simulink model "DR18E_Testpult"  (R2017a)
settings: Solver=ode1  StartTime=0.0  StopTime=Inf  FixedStep=0.001  RelTol=1e-3
PostLoadFcn:
  | , if any(exist('dsrtsu_mdlpostloadfcn', 'file') == [2, 3, 6]), try dsrtsu_mdlpostloadfcn('Execute', bdroot); catch fprintf('Error in PostLoadFcn (dsrtsu_mdlpostloadfcn) for model "%s":\n %s\n', bdroot, lasterr); end, end,
model workspace: external: MAT-File C:\Users\DeltaRacing\Documents\dSPACE\MABX_DR18E\Model\DR18E_MABX_Parameter.mat (data not in the file)
values from neighbouring files (symbols this model uses):
  am = 1/Ts    (= 1)    [DR18E_MABX_Parameter.m]
  bm = K/Ts    (= 0.05)    [DR18E_MABX_Parameter.m]
  cf = 41350    [DR18E_MABX_Parameter.m]
  cr = 41350    [DR18E_MABX_Parameter.m]
  Derating_HV_Battery_Kapa = 1    [DR18E_MABX_Parameter.m]
  Derating_Start_km = 16    [DR18E_MABX_Parameter.m]
  Drive_Mode = 0    [DR18E_MABX_Parameter.m]
  g = 1    [DR18E_MABX_Parameter.m]
  Gas_Modus = 2    [DR18E_MABX_Parameter.m]
  HV_Power_max = 80    [DR18E_MABX_Parameter.m]
  i_Getriebe = 3.3    [DR18E_MABX_Parameter.m]
  i_Lenkgetriebe = 4.32    [DR18E_MABX_Parameter.m]
  K_SET = 1    [DR18E_MABX_Parameter.m]
  Kapazitaet_HV_Battery_kWh = 6.6    [DR18E_MABX_Parameter.m]
  KW_T_Soll = 37    [DR18E_MABX_Parameter.m]
  lf = 1.2    [DR18E_MABX_Parameter.m]
  lr = 1.15    [DR18E_MABX_Parameter.m]
  m = mdriver + mvehicle    (= 310)    [DR18E_MABX_Parameter.m]
  M_max = 150    [DR18E_MABX_Parameter.m]
  Power_Limit_onoff = 0    [DR18E_MABX_Parameter.m]
  Reifenradius = 0.2351    [DR18E_MABX_Parameter.m]
  Strecke_Endu_km = 22    [DR18E_MABX_Parameter.m]
  TC_Decr_Gas = 0.00005    (= 5e-05)    [DR18E_MABX_Parameter.m]
  TC_Derivative = 0.4    [DR18E_MABX_Parameter.m]
  TC_Incr_Gas = 0.005    [DR18E_MABX_Parameter.m]
  TC_On = 0    [DR18E_MABX_Parameter.m]
  TC_Relay_Off = 0.065    [DR18E_MABX_Parameter.m]
  TC_Relay_On = 0.07    [DR18E_MABX_Parameter.m]
  TV_Mode = 2    [DR18E_MABX_Parameter.m]
  TV_On = 0    [DR18E_MABX_Parameter.m]
  TV_Override = 1    [DR18E_MABX_Parameter.m]
  y = 0.8    [DR18E_MABX_Parameter.m]
undefined symbols (not defined in the file or in its folder): D, DiscIntNeverNeededParam, I, K_OL, P
libraries: simulink x288, rtican x100, rtiusbflightreclib x40, rti1401lib_dio_type3 x10, simulink_extras x10, rti1401lib_adc_type4 x8, rti1401lib_II_base x7
(part 26 of 27)

== system DR18E_Testpult/Eingabe Fahrzeug/BMS/Voltage Stack 1-2/Voltage Stack 1/RX Timeout Detection2 ==
  RX status : Inport
  Timeout (n Samples) : Inport  Port=2
  Subsystem : Subsystem  TreatAsAtomicUnit=on
  Terminator_4 : Terminator
  RX Timeout Error : Outport
  wires:
  RX status/1 -> Subsystem/1(TXStatus)
  Subsystem/1(Rampe) -> Terminator_4/1
  Subsystem/2(RX Timeout Error) -> RX Timeout Error/1  "RX Timeout"
  Timeout (n Samples)/1 -> Subsystem/2(Timeout)

== system DR18E_Testpult/Eingabe Fahrzeug/BMS/Voltage Stack 1-2/Voltage Stack 2/RX Timeout Detection ==
  RX status : Inport
  Timeout (n Samples) : Inport  Port=2
  Subsystem : Subsystem  TreatAsAtomicUnit=on
  Terminator_4 : Terminator
  RX Timeout Error : Outport
  wires:
  RX status/1 -> Subsystem/1(TXStatus)
  Subsystem/1(Rampe) -> Terminator_4/1
  Subsystem/2(RX Timeout Error) -> RX Timeout Error/1  "RX Timeout"
  Timeout (n Samples)/1 -> Subsystem/2(Timeout)

== system DR18E_Testpult/Eingabe Fahrzeug/BMS/Voltage Stack 1-2/Voltage Stack 2/RX Timeout Detection1 ==
  RX status : Inport
  Timeout (n Samples) : Inport  Port=2
  Subsystem : Subsystem  TreatAsAtomicUnit=on
  Terminator_4 : Terminator
  RX Timeout Error : Outport
  wires:
  RX status/1 -> Subsystem/1(TXStatus)
  Subsystem/1(Rampe) -> Terminator_4/1
  Subsystem/2(RX Timeout Error) -> RX Timeout Error/1  "RX Timeout"
  Timeout (n Samples)/1 -> Subsystem/2(Timeout)

== system DR18E_Testpult/Eingabe Fahrzeug/BMS/Voltage Stack 1-2/Voltage Stack 2/RX Timeout Detection2 ==
  RX status : Inport
  Timeout (n Samples) : Inport  Port=2
  Subsystem : Subsystem  TreatAsAtomicUnit=on
  Terminator_4 : Terminator
  RX Timeout Error : Outport
  wires:
  RX status/1 -> Subsystem/1(TXStatus)
  Subsystem/1(Rampe) -> Terminator_4/1
  Subsystem/2(RX Timeout Error) -> RX Timeout Error/1  "RX Timeout"
  Timeout (n Samples)/1 -> Subsystem/2(Timeout)

== system DR18E_Testpult/Eingabe Fahrzeug/BMS/Voltage Stack 3-4/Voltage Stack 3/RX Timeout Detection ==
  RX status : Inport
  Timeout (n Samples) : Inport  Port=2
  Subsystem : Subsystem  TreatAsAtomicUnit=on
  Terminator_4 : Terminator
  RX Timeout Error : Outport
  wires:
  RX status/1 -> Subsystem/1(TXStatus)
  Subsystem/1(Rampe) -> Terminator_4/1
  Subsystem/2(RX Timeout Error) -> RX Timeout Error/1  "RX Timeout"
  Timeout (n Samples)/1 -> Subsystem/2(Timeout)

== system DR18E_Testpult/Eingabe Fahrzeug/BMS/Voltage Stack 3-4/Voltage Stack 3/RX Timeout Detection1 ==
  RX status : Inport
  Timeout (n Samples) : Inport  Port=2
  Subsystem : Subsystem  TreatAsAtomicUnit=on
  Terminator_4 : Terminator
  RX Timeout Error : Outport
  wires:
  RX status/1 -> Subsystem/1(TXStatus)
  Subsystem/1(Rampe) -> Terminator_4/1
  Subsystem/2(RX Timeout Error) -> RX Timeout Error/1  "RX Timeout"
  Timeout (n Samples)/1 -> Subsystem/2(Timeout)

== system DR18E_Testpult/Eingabe Fahrzeug/BMS/Voltage Stack 3-4/Voltage Stack 3/RX Timeout Detection2 ==
  RX status : Inport
  Timeout (n Samples) : Inport  Port=2
  Subsystem : Subsystem  TreatAsAtomicUnit=on
  Terminator_4 : Terminator
  RX Timeout Error : Outport
  wires:
  RX status/1 -> Subsystem/1(TXStatus)
  Subsystem/1(Rampe) -> Terminator_4/1
  Subsystem/2(RX Timeout Error) -> RX Timeout Error/1  "RX Timeout"
  Timeout (n Samples)/1 -> Subsystem/2(Timeout)

== system DR18E_Testpult/Eingabe Fahrzeug/BMS/Voltage Stack 3-4/Voltage Stack 4/RX Timeout Detection ==
  RX status : Inport
  Timeout (n Samples) : Inport  Port=2
  Subsystem : Subsystem  TreatAsAtomicUnit=on
  Terminator_4 : Terminator
  RX Timeout Error : Outport
  wires:
  RX status/1 -> Subsystem/1(TXStatus)
  Subsystem/1(Rampe) -> Terminator_4/1
  Subsystem/2(RX Timeout Error) -> RX Timeout Error/1  "RX Timeout"
  Timeout (n Samples)/1 -> Subsystem/2(Timeout)

== system DR18E_Testpult/Eingabe Fahrzeug/BMS/Voltage Stack 3-4/Voltage Stack 4/RX Timeout Detection1 ==
  RX status : Inport
  Timeout (n Samples) : Inport  Port=2
  Subsystem : Subsystem  TreatAsAtomicUnit=on
  Terminator_4 : Terminator
  RX Timeout Error : Outport
  wires:
  RX status/1 -> Subsystem/1(TXStatus)
  Subsystem/1(Rampe) -> Terminator_4/1
  Subsystem/2(RX Timeout Error) -> RX Timeout Error/1  "RX Timeout"
  Timeout (n Samples)/1 -> Subsystem/2(Timeout)

== system DR18E_Testpult/Eingabe Fahrzeug/BMS/Voltage Stack 3-4/Voltage Stack 4/RX Timeout Detection2 ==
  RX status : Inport
  Timeout (n Samples) : Inport  Port=2
  Subsystem : Subsystem  TreatAsAtomicUnit=on
  Terminator_4 : Terminator
  RX Timeout Error : Outport
  wires:
  RX status/1 -> Subsystem/1(TXStatus)
  Subsystem/1(Rampe) -> Terminator_4/1
  Subsystem/2(RX Timeout Error) -> RX Timeout Error/1  "RX Timeout"
  Timeout (n Samples)/1 -> Subsystem/2(Timeout)

== system DR18E_Testpult/Eingabe Fahrzeug/BMS/Voltage Stack 5-6/Voltage Stack 5/RX Timeout Detection ==
  RX status : Inport
  Timeout (n Samples) : Inport  Port=2
  Subsystem : Subsystem  TreatAsAtomicUnit=on
  Terminator_4 : Terminator
  RX Timeout Error : Outport
  wires:
  RX status/1 -> Subsystem/1(TXStatus)
  Subsystem/1(Rampe) -> Terminator_4/1
  Subsystem/2(RX Timeout Error) -> RX Timeout Error/1  "RX Timeout"
  Timeout (n Samples)/1 -> Subsystem/2(Timeout)

== system DR18E_Testpult/Eingabe Fahrzeug/BMS/Voltage Stack 5-6/Voltage Stack 5/RX Timeout Detection1 ==
  RX status : Inport
  Timeout (n Samples) : Inport  Port=2
  Subsystem : Subsystem  TreatAsAtomicUnit=on
  Terminator_4 : Terminator
  RX Timeout Error : Outport
  wires:
  RX status/1 -> Subsystem/1(TXStatus)
  Subsystem/1(Rampe) -> Terminator_4/1
  Subsystem/2(RX Timeout Error) -> RX Timeout Error/1  "RX Timeout"
  Timeout (n Samples)/1 -> Subsystem/2(Timeout)

== system DR18E_Testpult/Eingabe Fahrzeug/BMS/Voltage Stack 5-6/Voltage Stack 5/RX Timeout Detection2 ==
  RX status : Inport
  Timeout (n Samples) : Inport  Port=2
  Subsystem : Subsystem  TreatAsAtomicUnit=on
  Terminator_4 : Terminator
  RX Timeout Error : Outport
  wires:
  RX status/1 -> Subsystem/1(TXStatus)
  Subsystem/1(Rampe) -> Terminator_4/1
  Subsystem/2(RX Timeout Error) -> RX Timeout Error/1  "RX Timeout"
  Timeout (n Samples)/1 -> Subsystem/2(Timeout)

== system DR18E_Testpult/Eingabe Fahrzeug/BMS/Voltage Stack 5-6/Voltage Stack 6/RX Timeout Detection ==
  RX status : Inport
  Timeout (n Samples) : Inport  Port=2
  Subsystem : Subsystem  TreatAsAtomicUnit=on
  Terminator_4 : Terminator
  RX Timeout Error : Outport
  wires:
  RX status/1 -> Subsystem/1(TXStatus)
  Subsystem/1(Rampe) -> Terminator_4/1
  Subsystem/2(RX Timeout Error) -> RX Timeout Error/1  "RX Timeout"
  Timeout (n Samples)/1 -> Subsystem/2(Timeout)

== system DR18E_Testpult/Eingabe Fahrzeug/BMS/Voltage Stack 5-6/Voltage Stack 6/RX Timeout Detection1 ==
  RX status : Inport
  Timeout (n Samples) : Inport  Port=2
  Subsystem : Subsystem  TreatAsAtomicUnit=on
  Terminator_4 : Terminator
  RX Timeout Error : Outport
  wires:
  RX status/1 -> Subsystem/1(TXStatus)
  Subsystem/1(Rampe) -> Terminator_4/1
  Subsystem/2(RX Timeout Error) -> RX Timeout Error/1  "RX Timeout"
  Timeout (n Samples)/1 -> Subsystem/2(Timeout)

== system DR18E_Testpult/Eingabe Fahrzeug/BMS/Voltage Stack 5-6/Voltage Stack 6/RX Timeout Detection2 ==
  RX status : Inport
  Timeout (n Samples) : Inport  Port=2
  Subsystem : Subsystem  TreatAsAtomicUnit=on
  Terminator_4 : Terminator
  RX Timeout Error : Outport
  wires:
  RX status/1 -> Subsystem/1(TXStatus)
  Subsystem/1(Rampe) -> Terminator_4/1
  Subsystem/2(RX Timeout Error) -> RX Timeout Error/1  "RX Timeout"
  Timeout (n Samples)/1 -> Subsystem/2(Timeout)

== system DR18E_Testpult/Eingabe Fahrzeug/BMS/Voltage Stack 7-8/Voltage Stack 7/RX Timeout Detection ==
  RX status : Inport
  Timeout (n Samples) : Inport  Port=2
  Subsystem : Subsystem  TreatAsAtomicUnit=on
  Terminator_4 : Terminator
  RX Timeout Error : Outport
  wires:
  RX status/1 -> Subsystem/1(TXStatus)
  Subsystem/1(Rampe) -> Terminator_4/1
  Subsystem/2(RX Timeout Error) -> RX Timeout Error/1  "RX Timeout"
  Timeout (n Samples)/1 -> Subsystem/2(Timeout)

== system DR18E_Testpult/Eingabe Fahrzeug/BMS/Voltage Stack 7-8/Voltage Stack 7/RX Timeout Detection1 ==
  RX status : Inport
  Timeout (n Samples) : Inport  Port=2
  Subsystem : Subsystem  TreatAsAtomicUnit=on
  Terminator_4 : Terminator
  RX Timeout Error : Outport
  wires:
  RX status/1 -> Subsystem/1(TXStatus)
  Subsystem/1(Rampe) -> Terminator_4/1
  Subsystem/2(RX Timeout Error) -> RX Timeout Error/1  "RX Timeout"
  Timeout (n Samples)/1 -> Subsystem/2(Timeout)

== system DR18E_Testpult/Eingabe Fahrzeug/BMS/Voltage Stack 7-8/Voltage Stack 7/RX Timeout Detection2 ==
  RX status : Inport
  Timeout (n Samples) : Inport  Port=2
  Subsystem : Subsystem  TreatAsAtomicUnit=on
  Terminator_4 : Terminator
  RX Timeout Error : Outport
  wires:
  RX status/1 -> Subsystem/1(TXStatus)
  Subsystem/1(Rampe) -> Terminator_4/1
  Subsystem/2(RX Timeout Error) -> RX Timeout Error/1  "RX Timeout"
  Timeout (n Samples)/1 -> Subsystem/2(Timeout)

== system DR18E_Testpult/Eingabe Fahrzeug/BMS/Voltage Stack 7-8/Voltage Stack 8/RX Timeout Detection ==
  RX status : Inport
  Timeout (n Samples) : Inport  Port=2
  Subsystem : Subsystem  TreatAsAtomicUnit=on
  Terminator_4 : Terminator
  RX Timeout Error : Outport
  wires:
  RX status/1 -> Subsystem/1(TXStatus)
  Subsystem/1(Rampe) -> Terminator_4/1
  Subsystem/2(RX Timeout Error) -> RX Timeout Error/1  "RX Timeout"
  Timeout (n Samples)/1 -> Subsystem/2(Timeout)

== system DR18E_Testpult/Eingabe Fahrzeug/BMS/Voltage Stack 7-8/Voltage Stack 8/RX Timeout Detection1 ==
  RX status : Inport
  Timeout (n Samples) : Inport  Port=2
  Subsystem : Subsystem  TreatAsAtomicUnit=on
  Terminator_4 : Terminator
  RX Timeout Error : Outport
  wires:
  RX status/1 -> Subsystem/1(TXStatus)
  Subsystem/1(Rampe) -> Terminator_4/1
  Subsystem/2(RX Timeout Error) -> RX Timeout Error/1  "RX Timeout"
  Timeout (n Samples)/1 -> Subsystem/2(Timeout)

== system DR18E_Testpult/Eingabe Fahrzeug/BMS/Voltage Stack 7-8/Voltage Stack 8/RX Timeout Detection2 ==
  RX status : Inport
  Timeout (n Samples) : Inport  Port=2
  Subsystem : Subsystem  TreatAsAtomicUnit=on
  Terminator_4 : Terminator
  RX Timeout Error : Outport
  wires:
  RX status/1 -> Subsystem/1(TXStatus)
  Subsystem/1(Rampe) -> Terminator_4/1
  Subsystem/2(RX Timeout Error) -> RX Timeout Error/1  "RX Timeout"
  Timeout (n Samples)/1 -> Subsystem/2(Timeout)

== system DR18E_Testpult/Eingabe Fahrzeug/Inverter Feedback Messages/Istwerte Umrichter 1 empfangen /Drehzahl/PT1 Discrete2 ==
  u : Inport
  K : Inport  Port=2
  T : Inport  Port=3
  Memory : Memory
  Product : Product
  Product1 : Product
  Subsystem : Subsystem
  Sum : Sum  Inputs=|+-
  Sum1 : Sum  Inputs=|++
  y : Outport
  wires:
  K/1 -> Product/1
  Subsystem/1(T*) -> Product1/1
  u/1 -> Product/2
  Sum/1 -> Product1/2
  Product1/1 -> Sum1/1
  Memory/1 -> Sum1/2, Sum/2
  Sum1/1 -> y/1, Memory/1
  Product/1 -> Sum/1
  T/1 -> Subsystem/1(T)

== system DR18E_Testpult/Eingabe Fahrzeug/Inverter Feedback Messages/Istwerte Umrichter 1 empfangen /Drehzahl/Skalierung Drehzahl ==
  In1 : Inport
  Gain : Gain  Gain=4000/2^15
  Out1 : Outport
  wires:
  Gain/1 -> Out1/1
  In1/1 -> Gain/1

== system DR18E_Testpult/Eingabe Fahrzeug/Inverter Feedback Messages/Istwerte Umrichter 2 empfangen/Drehzahl/PT1 Discrete2 ==
  u : Inport
  K : Inport  Port=2
  T : Inport  Port=3
  Memory : Memory
  Product : Product
  Product1 : Product
  Subsystem : Subsystem
  Sum : Sum  Inputs=|+-
  Sum1 : Sum  Inputs=|++
  y : Outport
  wires:
  K/1 -> Product/1
  Subsystem/1(T*) -> Product1/1
  u/1 -> Product/2
  Sum/1 -> Product1/2
  Product1/1 -> Sum1/1
  Memory/1 -> Sum1/2, Sum/2
  Sum1/1 -> y/1, Memory/1
  Product/1 -> Sum/1
  T/1 -> Subsystem/1(T)

== system DR18E_Testpult/Eingabe Fahrzeug/Inverter Feedback Messages/Istwerte Umrichter 2 empfangen/Drehzahl/Skalierung Drehzahl ==
  In1 : Inport
  Gain : Gain  Gain=4000/(2^15)
  Out1 : Outport
  wires:
  In1/1 -> Gain/1
  Gain/1 -> Out1/1

== system DR18E_Testpult/Eingabe Fahrzeug/MicroAutoBox/AI/Umrechnung Widerstand - Temperatur NTC/PT1 Discrete1 ==
  u : Inport
  K : Inport  Port=2
  T : Inport  Port=3
  Memory : Memory
  Product : Product
  Product1 : Product
  Subsystem : Subsystem
  Sum : Sum  Inputs=|+-
  Sum1 : Sum  Inputs=|++
  y : Outport
  wires:
  K/1 -> Product/1
  Subsystem/1(T*) -> Product1/1
  u/1 -> Product/2
  Sum/1 -> Product1/2
  Product1/1 -> Sum1/1
  Memory/1 -> Sum1/2, Sum/2
  Sum1/1 -> y/1, Memory/1
  Product/1 -> Sum/1
  T/1 -> Subsystem/1(T)

== system DR18E_Testpult/Eingabe Fahrzeug/MicroAutoBox/AI/Umrechnung Widerstand - Temperatur NTC1/PT1 Discrete1 ==
  u : Inport
  K : Inport  Port=2
  T : Inport  Port=3
  Memory : Memory
  Product : Product
  Product1 : Product
  Subsystem : Subsystem
  Sum : Sum  Inputs=|+-
  Sum1 : Sum  Inputs=|++
  y : Outport
  wires:
  K/1 -> Product/1
  Subsystem/1(T*) -> Product1/1
  u/1 -> Product/2
  Sum/1 -> Product1/2
  Product1/1 -> Sum1/1
  Memory/1 -> Sum1/2, Sum/2
  Sum1/1 -> y/1, Memory/1
  Product/1 -> Sum/1
  T/1 -> Subsystem/1(T)

== system DR18E_Testpult/RTI Data/RTI Data Store/RTI Data Store/RTI Data Store/RTI Data Store ==

== system DR18E_Testpult/Verarbeitung/Bremse/PlausibilityCheck/PT1 Discrete1/Subsystem ==
  T : Inport
  Constant : Constant
  Constant2 : Constant
  Divide : Product  Inputs=*/
  Divide1 : Product  Inputs=*/
  Sum : Sum  Inputs=|++
  Weighted Sample Time : SampleTimeMath  TsampMathOp=Ts Only
  T* : Outport
  wires:
  Divide/1 -> T*/1
  Weighted Sample Time/1 -> Divide1/2
  Constant/1 -> Divide/1
  Sum/1 -> Divide/2
  T/1 -> Divide1/1
  Constant2/1 -> Sum/2
  Divide1/1 -> Sum/1

== system DR18E_Testpult/Verarbeitung/DR18E Torque Control/Derating/Derating_Strategie_Reichweite/Verbrauch_Wh//km ==
  In1 : Inport
  Data Type Conversion : DataTypeConversion
  Gain : Gain
  USB_FLIGHT_REC_BL1 : rtiusbflightreclib/USB_FLIGHT_REC_BL1  VarName=Verbrauch_Whprokm  DataType=Single  SampleTime=-1  TLCFileName=rtiusbflightrecwrite  Reserved1=[]  Reserved2=[]  Reserved3=[]  Reserved4=[]  DSProperties=struct('RTI',struct('Version',uint32(3),'BlockType',struct('isSLSource',uint8(0),'isSLSink',uint8(1),'isHWSource',uint8(0),'isHWSink',uint8(0),'isSetup',uint8(0),'isInline',uint8(1),'isNonInline',uint8(0),'isInterrupt',uint8(0),'isChannelwise',uint8(0)),'IOBoardType',{{'DSUSB','FLIGHTREC'}},'UnitType','FLIGHTREC','Identifier','WRITE','DialogType','SL','BlockSet','RTIUSBFLIGHTREC','SlaveProcessor','NONE'))  RTIBlockInterface=struct('InputPortsActive',1,'InputPortsWidth',int32(1),'InputPortsDataType',{{'SS_SINGLE'}},'BlockDisplay',{{['Write to\nUSB Flight Recorder'],'center'}},'IconTransparency','off','InitLevel',3,'BlockName',struct('Token',{{'USB_FLIGHT_REC_BL1'}}),'MaskDescription',['Write input to the Flight Recorder. Recorded data can be referenced by the specified variable.'],'SampleTime',{{-1}})  RTIBlockParameters=struct('VarName',{{'Verbrauch_Whprokm','OFF',[]}},'DataType',{{'Single','OFF',[]}},'SampleTime',{{-1,'OFF',[]}},'TLCFileName',{{'rtiusbflightrecwrite','OFF',[]}})  RTISFcnParameters=struct('VarName','char','DataType','char','SampleTime','double','TLCFileName','char')  RTIBlockParaDefault=struct('VarName','Var1','DataType','Single','SampleTime',-1,'TLCFileName','rtiusbflightrecwrite')
      settings: SourceProductName=dSPACE RTI USB Flight Rec Blockset
  wires:
  Data Type Conversion/1 -> USB_FLIGHT_REC_BL1/1
  In1/1 -> Gain/1
  Gain/1 -> Data Type Conversion/1

== system DR18E_Testpult/Verarbeitung/DR18E Torque Control/TV RL/TV DR17E/Drehmomentverteilung links//rechts ==
  DeltaM_in : Inport
  Gain links : Gain
  deltaM_Out : Outport
  wires:
  DeltaM_in/1 -> Gain links/1  "delta_ML"
  Gain links/1 -> deltaM_Out/1

== system DR18E_Testpult/Verarbeitung/DR18E Torque Control/TV RL/TV DR17E/Ermittlung Sollgierrate ==
  vx-ms : Inport
  Radeinschlagwinkel-deg : Inport  Port=2
  Divide : Product  Inputs=*/
  EG Einlenkgradient : Constant  Value=0.0025
  Product : Product
  Product1 : Product
  Sum : Sum  Inputs=|++
  Sum1 : Sum  Inputs=+
  Tapped Delay : simulink/Discrete/Tapped Delay  vinit=0.0  samptime=-1  NumDelays=5  DelayOrder=Oldest  includeCurrent=off
  deg-rad : Gain  Gain=2*pi/360
  deg-rad1 : Gain  Gain=1/5
  l Radstand : Constant  Value=1.53
  rad-deg : Gain  Gain=360/(2*pi)
  sqr : Math  Operator=square  SaturateOnIntegerOverflow=on
  Psipunkt-Soll-deg-s : Outport
  wires:
  rad-deg/1 -> Psipunkt-Soll-deg-s/1
  Radeinschlagwinkel-deg/1 -> deg-rad/1
  sqr/1 -> Product1/1
  EG Einlenkgradient/1 -> Product1/2
  Product1/1 -> Sum/1
  l Radstand/1 -> Sum/2
  vx-ms/1 -> sqr/1, Product/2
  deg-rad/1 -> Product/1
  Product/1 -> Divide/1
  Sum/1 -> Divide/2
  Divide/1 -> rad-deg/1
  Tapped Delay/1 -> deg-rad1/1

== system DR18E_Testpult/Verarbeitung/DR18E Torque Control/TV RL/TV DR17E/FlightRecorder4 ==
  In1 : Inport
  Data Type Conversion : DataTypeConversion
  Gain : Gain
  USB_FLIGHT_REC_BL1 : rtiusbflightreclib/USB_FLIGHT_REC_BL1  VarName=PsiPunktSoll  DataType=Single  SampleTime=-1  TLCFileName=rtiusbflightrecwrite  Reserved1=[]  Reserved2=[]  Reserved3=[]  Reserved4=[]  DSProperties=struct('RTI',struct('Version',uint32(3),'BlockType',struct('isSLSource',uint8(0),'isSLSink',uint8(1),'isHWSource',uint8(0),'isHWSink',uint8(0),'isSetup',uint8(0),'isInline',uint8(1),'isNonInline',uint8(0),'isInterrupt',uint8(0),'isChannelwise',uint8(0)),'IOBoardType',{{'DSUSB','FLIGHTREC'}},'UnitType','FLIGHTREC','Identifier','WRITE','DialogType','SL','BlockSet','RTIUSBFLIGHTREC','SlaveProcessor','NONE'))  RTIBlockInterface=struct('InputPortsActive',1,'InputPortsWidth',int32(1),'InputPortsDataType',{{'SS_SINGLE'}},'BlockDisplay',{{['Write to\nUSB Flight Recorder'],'center'}},'IconTransparency','off','InitLevel',3,'BlockName',struct('Token',{{'USB_FLIGHT_REC_BL1'}}),'MaskDescription',['Write input to the Flight Recorder. Recorded data can be referenced by the specified variable.'],'SampleTime',{{-1}})  RTIBlockParameters=struct('VarName',{{'PsiPunktSoll','OFF',[]}},'DataType',{{'Single','OFF',[]}},'SampleTime',{{-1,'OFF',[]}},'TLCFileName',{{'rtiusbflightrecwrite','OFF',[]}})  RTISFcnParameters=struct('VarName','char','DataType','char','SampleTime','double','TLCFileName','char')  RTIBlockParaDefault=struct('VarName','Var1','DataType','Single','SampleTime',-1,'TLCFileName','rtiusbflightrecwrite')
      settings: SourceProductName=dSPACE RTI USB Flight Rec Blockset
  wires:
  Data Type Conversion/1 -> USB_FLIGHT_REC_BL1/1
  In1/1 -> Gain/1
  Gain/1 -> Data Type Conversion/1

== system DR18E_Testpult/Verarbeitung/DR18E Torque Control/TV RL/TV DR17E/Vorsteuerung+PID ==
  note: 0.25
  PsiPunktSoll : Inport
  PsiPunktIst : Inport  Port=2
  2*Jz*rdyn/(br*i) : Gain  Gain=2*105.33*0.228/(1.15*1.8)
  Constant : Constant  Value=0
  K_ClosedLoop : Gain
  K_OpenLoop : Gain  Commented=on  Gain=K_OL
  K_OpenLoop1 : Gain  Gain=0.25
  Manual Switch : ManualSwitch  CurrentSetting=0
  PID : simulink/Continuous/PID Controller  Commented=on  Controller=PID  TimeDomain=Discrete-time  SampleTime=0.01  IntegratorMethod=Forward Euler  FilterMethod=Forward Euler  Form=Parallel  UseFilter=on  ControllerParametersSource=internal  P=P  I=I  D=D  N=127  InitialConditionSource=internal  InitialConditionForIntegrator=0  InitialConditionForFilter=0  ExternalReset=none  LimitOutput=off  UpperSaturationLimit=inf  LowerSaturationLimit=-inf  LinearizeAsGain=off  AntiWindupMode=none  Kb=1  TrackingMode=off  Kt=1  PParamMin=[]  PParamMax=[]  IParamMin=[]  IParamMax=[]  DParamMin=[]  DParamMax=[]  NParamMin=[]  NParamMax=[]  KbParamMin=[]  KbParamMax=[]  KtParamMin=[]  KtParamMax=[]  POutMin=[]  POutMax=[]  IOutMin=[]  IOutMax=[]  DOutMin=[]  DOutMax=[]  NOutMin=[]  NOutMax=[]  KbOutMin=[]  KbOutMax=[]  KtOutMin=[]  KtOutMax=[]  IntegratorOutMin=[]  IntegratorOutMax=[]  FilterOutMin=[]  FilterOutMax=[]  SumOutMin=[]  SumOutMax=[]  SumI1OutMin=[]  SumI1OutMax=[]  SumI2OutMin=[]  SumI2OutMax=[]  SumI3OutMin=[]  SumI3OutMax=[]  SumDOutMin=[]  SumDOutMax=[]  SaturationOutMin=[]  SaturationOutMax=[]  IntegratorContinuousStateAttributes=''  IntegratorStateMustResolveToSignalObject=off  IntegratorRTWStateStorageClass=Auto  FilterContinuousStateAttributes=''  FilterStateMustResolveToSignalObject=off  FilterRTWStateStorageClass=Auto  DifferentiatorICPrevScaledInput=0  DifferentiatorOutMin=[]  DifferentiatorOutMax=[]  InitialConditionSetting=State (most efficient)
  PID_fromGA : simulink/Continuous/PID Controller  Controller=PID  TimeDomain=Discrete-time  SampleTime=0.01  IntegratorMethod=Forward Euler  FilterMethod=Forward Euler  Form=Parallel  UseFilter=on  ControllerParametersSource=internal  P=0.6557  I=0.0344  D=0.5853  N=127  InitialConditionSource=internal  InitialConditionForIntegrator=0  InitialConditionForFilter=0  ExternalReset=none  LimitOutput=off  UpperSaturationLimit=inf  LowerSaturationLimit=-inf  LinearizeAsGain=off  AntiWindupMode=none  Kb=1  TrackingMode=off  Kt=1  PParamMin=[]  PParamMax=[]  IParamMin=[]  IParamMax=[]  DParamMin=[]  DParamMax=[]  NParamMin=[]  NParamMax=[]  KbParamMin=[]  KbParamMax=[]  KtParamMin=[]  KtParamMax=[]  POutMin=[]  POutMax=[]  IOutMin=[]  IOutMax=[]  DOutMin=[]  DOutMax=[]  NOutMin=[]  NOutMax=[]  KbOutMin=[]  KbOutMax=[]  KtOutMin=[]  KtOutMax=[]  IntegratorOutMin=[]  IntegratorOutMax=[]  FilterOutMin=[]  FilterOutMax=[]  SumOutMin=[]  SumOutMax=[]  SumI1OutMin=[]  SumI1OutMax=[]  SumI2OutMin=[]  SumI2OutMax=[]  SumI3OutMin=[]  SumI3OutMax=[]  SumDOutMin=[]  SumDOutMax=[]  SaturationOutMin=[]  SaturationOutMax=[]  IntegratorContinuousStateAttributes=''  IntegratorStateMustResolveToSignalObject=off  IntegratorRTWStateStorageClass=Auto  FilterContinuousStateAttributes=''  FilterStateMustResolveToSignalObject=off  FilterRTWStateStorageClass=Auto  DifferentiatorICPrevScaledInput=0  DifferentiatorOutMin=[]  DifferentiatorOutMax=[]  InitialConditionSetting=State (most efficient)
  PID_fromOptim : simulink/Continuous/PID Controller  Controller=PID  TimeDomain=Discrete-time  SampleTime=0.01  IntegratorMethod=Forward Euler  FilterMethod=Forward Euler  Form=Parallel  UseFilter=on  ControllerParametersSource=internal  P=0.5164  I=2.5714  D=1.7405  N=127  InitialConditionSource=internal  InitialConditionForIntegrator=0  InitialConditionForFilter=0  ExternalReset=none  LimitOutput=off  UpperSaturationLimit=inf  LowerSaturationLimit=-inf  LinearizeAsGain=off  AntiWindupMode=none  Kb=1  TrackingMode=off  Kt=1  PParamMin=[]  PParamMax=[]  IParamMin=[]  IParamMax=[]  DParamMin=[]  DParamMax=[]  NParamMin=[]  NParamMax=[]  KbParamMin=[]  KbParamMax=[]  KtParamMin=[]  KtParamMax=[]  POutMin=[]  POutMax=[]  IOutMin=[]  IOutMax=[]  DOutMin=[]  DOutMax=[]  NOutMin=[]  NOutMax=[]  KbOutMin=[]  KbOutMax=[]  KtOutMin=[]  KtOutMax=[]  IntegratorOutMin=[]  IntegratorOutMax=[]  FilterOutMin=[]  FilterOutMax=[]  SumOutMin=[]  SumOutMax=[]  SumI1OutMin=[]  SumI1OutMax=[]  SumI2OutMin=[]  SumI2OutMax=[]  SumI3OutMin=[]  SumI3OutMax=[]  SumDOutMin=[]  SumDOutMax=[]  SaturationOutMin=[]  SaturationOutMax=[]  IntegratorContinuousStateAttributes=''  IntegratorStateMustResolveToSignalObject=off  IntegratorRTWStateStorageClass=Auto  FilterContinuousStateAttributes=''  FilterStateMustResolveToSignalObject=off  FilterRTWStateStorageClass=Auto  DifferentiatorICPrevScaledInput=0  DifferentiatorOutMin=[]  DifferentiatorOutMax=[]  InitialConditionSetting=State (most efficient)
  PID_from_BJ : simulink/Continuous/PID Controller  Controller=PID  TimeDomain=Discrete-time  SampleTime=0.01  IntegratorMethod=Forward Euler  FilterMethod=Forward Euler  Form=Parallel  UseFilter=on  ControllerParametersSource=internal  P=8.4755768690941  I=0  D=-0.329825259958135  N=18.7162193324192  InitialConditionSource=internal  InitialConditionForIntegrator=0  InitialConditionForFilter=0  ExternalReset=none  LimitOutput=off  UpperSaturationLimit=inf  LowerSaturationLimit=-inf  LinearizeAsGain=off  AntiWindupMode=none  Kb=1  TrackingMode=off  Kt=1  PParamMin=[]  PParamMax=[]  IParamMin=[]  IParamMax=[]  DParamMin=[]  DParamMax=[]  NParamMin=[]  NParamMax=[]  KbParamMin=[]  KbParamMax=[]  KtParamMin=[]  KtParamMax=[]  POutMin=[]  POutMax=[]  IOutMin=[]  IOutMax=[]  DOutMin=[]  DOutMax=[]  NOutMin=[]  NOutMax=[]  KbOutMin=[]  KbOutMax=[]  KtOutMin=[]  KtOutMax=[]  IntegratorOutMin=[]  IntegratorOutMax=[]  FilterOutMin=[]  FilterOutMax=[]  SumOutMin=[]  SumOutMax=[]  SumI1OutMin=[]  SumI1OutMax=[]  SumI2OutMin=[]  SumI2OutMax=[]  SumI3OutMin=[]  SumI3OutMax=[]  SumDOutMin=[]  SumDOutMax=[]  SaturationOutMin=[]  SaturationOutMax=[]  IntegratorContinuousStateAttributes=''  IntegratorStateMustResolveToSignalObject=off  IntegratorRTWStateStorageClass=Auto  FilterContinuousStateAttributes=''  FilterStateMustResolveToSignalObject=off  FilterRTWStateStorageClass=Auto  DifferentiatorICPrevScaledInput=0  DifferentiatorOutMin=[]  DifferentiatorOutMax=[]  InitialConditionSetting=State (most efficient)
  Rate Transition : RateTransition
  Rate Transition1 : RateTransition
  Sum : Sum  Inputs=|+-
  Sum1 : Sum  Inputs=+|+
  DeltaM : Outport
  wires:
  PsiPunktIst/1 -> Sum/2
  PsiPunktSoll/1 -> Sum/1
  Sum/1 -> Rate Transition/1
  2*Jz*rdyn/(br*i)/1 -> Sum1/1
  Manual Switch/1 -> Sum1/2
  Sum1/1 -> Rate Transition1/1
  Rate Transition/1 -> K_OpenLoop1/1, K_ClosedLoop/1
  Rate Transition1/1 -> DeltaM/1
  Constant/1 -> Manual Switch/2
  K_OpenLoop1/1 -> 2*Jz*rdyn/(br*i)/1
  K_ClosedLoop/1 -> PID_fromGA/1
  PID_fromGA/1 -> Manual Switch/1

== system DR18E_Testpult/Verarbeitung/DR18E Torque Control/TV RR/TV DR17E/Drehmomentverteilung links//rechts ==
  DeltaM_in : Inport
  Gain rechts : Gain
  deltaM_Out : Outport
  wires:
  DeltaM_in/1 -> Gain rechts/1  "delta_ML"
  Gain rechts/1 -> deltaM_Out/1

== system DR18E_Testpult/Verarbeitung/DR18E Torque Control/TV RR/TV DR17E/Ermittlung Sollgierrate ==
  vx-ms : Inport
  Radeinschlagwinkel-deg : Inport  Port=2
  Divide : Product  Inputs=*/
  EG Einlenkgradient : Constant  Value=0.0025
  Product : Product
  Product1 : Product
  Sum : Sum  Inputs=|++
  Sum1 : Sum  Inputs=+
  Tapped Delay : simulink/Discrete/Tapped Delay  vinit=0.0  samptime=-1  NumDelays=5  DelayOrder=Oldest  includeCurrent=off
  deg-rad : Gain  Gain=2*pi/360
  deg-rad1 : Gain  Gain=1/5
  l Radstand : Constant  Value=1.53
  rad-deg : Gain  Gain=360/(2*pi)
  sqr : Math  Operator=square  SaturateOnIntegerOverflow=on
  Psipunkt-Soll-deg-s : Outport
  wires:
  rad-deg/1 -> Psipunkt-Soll-deg-s/1
  Radeinschlagwinkel-deg/1 -> deg-rad/1
  sqr/1 -> Product1/1
  EG Einlenkgradient/1 -> Product1/2
  Product1/1 -> Sum/1
  l Radstand/1 -> Sum/2
  vx-ms/1 -> sqr/1, Product/2
  deg-rad/1 -> Product/1
  Product/1 -> Divide/1
  Sum/1 -> Divide/2
  Divide/1 -> rad-deg/1
  Tapped Delay/1 -> deg-rad1/1

== system DR18E_Testpult/Verarbeitung/DR18E Torque Control/TV RR/TV DR17E/FlightRecorder4 ==
  In1 : Inport
  Data Type Conversion : DataTypeConversion
  Gain : Gain
  USB_FLIGHT_REC_BL1 : rtiusbflightreclib/USB_FLIGHT_REC_BL1  VarName=PsiPunktSoll2  DataType=Single  SampleTime=-1  TLCFileName=rtiusbflightrecwrite  Reserved1=[]  Reserved2=[]  Reserved3=[]  Reserved4=[]  DSProperties=struct('RTI',struct('Version',uint32(3),'BlockType',struct('isSLSource',uint8(0),'isSLSink',uint8(1),'isHWSource',uint8(0),'isHWSink',uint8(0),'isSetup',uint8(0),'isInline',uint8(1),'isNonInline',uint8(0),'isInterrupt',uint8(0),'isChannelwise',uint8(0)),'IOBoardType',{{'DSUSB','FLIGHTREC'}},'UnitType','FLIGHTREC','Identifier','WRITE','DialogType','SL','BlockSet','RTIUSBFLIGHTREC','SlaveProcessor','NONE'))  RTIBlockInterface=struct('InputPortsActive',1,'InputPortsWidth',int32(1),'InputPortsDataType',{{'SS_SINGLE'}},'BlockDisplay',{{['Write to\nUSB Flight Recorder'],'center'}},'IconTransparency','off','InitLevel',3,'BlockName',struct('Token',{{'USB_FLIGHT_REC_BL1'}}),'MaskDescription',['Write input to the Flight Recorder. Recorded data can be referenced by the specified variable.'],'SampleTime',{{-1}})  RTIBlockParameters=struct('VarName',{{'PsiPunktSoll2','OFF',[]}},'DataType',{{'Single','OFF',[]}},'SampleTime',{{-1,'OFF',[]}},'TLCFileName',{{'rtiusbflightrecwrite','OFF',[]}})  RTISFcnParameters=struct('VarName','char','DataType','char','SampleTime','double','TLCFileName','char')  RTIBlockParaDefault=struct('VarName','Var1','DataType','Single','SampleTime',-1,'TLCFileName','rtiusbflightrecwrite')
      settings: SourceProductName=dSPACE RTI USB Flight Rec Blockset
  wires:
  Data Type Conversion/1 -> USB_FLIGHT_REC_BL1/1
  In1/1 -> Gain/1
  Gain/1 -> Data Type Conversion/1

== system DR18E_Testpult/Verarbeitung/DR18E Torque Control/TV RR/TV DR17E/Vorsteuerung+PID ==
  note: 0.25
  PsiPunktSoll : Inport
  PsiPunktIst : Inport  Port=2
  2*Jz*rdyn/(br*i) : Gain  Gain=2*105.33*0.228/(1.15*1.8)
  Constant : Constant  Value=0
  K_ClosedLoop : Gain
  K_OpenLoop : Gain  Commented=on  Gain=K_OL
  K_OpenLoop1 : Gain  Gain=0.25
  Manual Switch : ManualSwitch  CurrentSetting=0
  PID : simulink/Continuous/PID Controller  Commented=on  Controller=PID  TimeDomain=Discrete-time  SampleTime=0.01  IntegratorMethod=Forward Euler  FilterMethod=Forward Euler  Form=Parallel  UseFilter=on  ControllerParametersSource=internal  P=P  I=I  D=D  N=127  InitialConditionSource=internal  InitialConditionForIntegrator=0  InitialConditionForFilter=0  ExternalReset=none  LimitOutput=off  UpperSaturationLimit=inf  LowerSaturationLimit=-inf  LinearizeAsGain=off  AntiWindupMode=none  Kb=1  TrackingMode=off  Kt=1  PParamMin=[]  PParamMax=[]  IParamMin=[]  IParamMax=[]  DParamMin=[]  DParamMax=[]  NParamMin=[]  NParamMax=[]  KbParamMin=[]  KbParamMax=[]  KtParamMin=[]  KtParamMax=[]  POutMin=[]  POutMax=[]  IOutMin=[]  IOutMax=[]  DOutMin=[]  DOutMax=[]  NOutMin=[]  NOutMax=[]  KbOutMin=[]  KbOutMax=[]  KtOutMin=[]  KtOutMax=[]  IntegratorOutMin=[]  IntegratorOutMax=[]  FilterOutMin=[]  FilterOutMax=[]  SumOutMin=[]  SumOutMax=[]  SumI1OutMin=[]  SumI1OutMax=[]  SumI2OutMin=[]  SumI2OutMax=[]  SumI3OutMin=[]  SumI3OutMax=[]  SumDOutMin=[]  SumDOutMax=[]  SaturationOutMin=[]  SaturationOutMax=[]  IntegratorContinuousStateAttributes=''  IntegratorStateMustResolveToSignalObject=off  IntegratorRTWStateStorageClass=Auto  FilterContinuousStateAttributes=''  FilterStateMustResolveToSignalObject=off  FilterRTWStateStorageClass=Auto  DifferentiatorICPrevScaledInput=0  DifferentiatorOutMin=[]  DifferentiatorOutMax=[]  InitialConditionSetting=State (most efficient)
  PID_fromGA : simulink/Continuous/PID Controller  Controller=PID  TimeDomain=Discrete-time  SampleTime=0.01  IntegratorMethod=Forward Euler  FilterMethod=Forward Euler  Form=Parallel  UseFilter=on  ControllerParametersSource=internal  P=0.6557  I=0.0344  D=0.5853  N=127  InitialConditionSource=internal  InitialConditionForIntegrator=0  InitialConditionForFilter=0  ExternalReset=none  LimitOutput=off  UpperSaturationLimit=inf  LowerSaturationLimit=-inf  LinearizeAsGain=off  AntiWindupMode=none  Kb=1  TrackingMode=off  Kt=1  PParamMin=[]  PParamMax=[]  IParamMin=[]  IParamMax=[]  DParamMin=[]  DParamMax=[]  NParamMin=[]  NParamMax=[]  KbParamMin=[]  KbParamMax=[]  KtParamMin=[]  KtParamMax=[]  POutMin=[]  POutMax=[]  IOutMin=[]  IOutMax=[]  DOutMin=[]  DOutMax=[]  NOutMin=[]  NOutMax=[]  KbOutMin=[]  KbOutMax=[]  KtOutMin=[]  KtOutMax=[]  IntegratorOutMin=[]  IntegratorOutMax=[]  FilterOutMin=[]  FilterOutMax=[]  SumOutMin=[]  SumOutMax=[]  SumI1OutMin=[]  SumI1OutMax=[]  SumI2OutMin=[]  SumI2OutMax=[]  SumI3OutMin=[]  SumI3OutMax=[]  SumDOutMin=[]  SumDOutMax=[]  SaturationOutMin=[]  SaturationOutMax=[]  IntegratorContinuousStateAttributes=''  IntegratorStateMustResolveToSignalObject=off  IntegratorRTWStateStorageClass=Auto  FilterContinuousStateAttributes=''  FilterStateMustResolveToSignalObject=off  FilterRTWStateStorageClass=Auto  DifferentiatorICPrevScaledInput=0  DifferentiatorOutMin=[]  DifferentiatorOutMax=[]  InitialConditionSetting=State (most efficient)
  PID_fromOptim : simulink/Continuous/PID Controller  Controller=PID  TimeDomain=Discrete-time  SampleTime=0.01  IntegratorMethod=Forward Euler  FilterMethod=Forward Euler  Form=Parallel  UseFilter=on  ControllerParametersSource=internal  P=0.5164  I=2.5714  D=1.7405  N=127  InitialConditionSource=internal  InitialConditionForIntegrator=0  InitialConditionForFilter=0  ExternalReset=none  LimitOutput=off  UpperSaturationLimit=inf  LowerSaturationLimit=-inf  LinearizeAsGain=off  AntiWindupMode=none  Kb=1  TrackingMode=off  Kt=1  PParamMin=[]  PParamMax=[]  IParamMin=[]  IParamMax=[]  DParamMin=[]  DParamMax=[]  NParamMin=[]  NParamMax=[]  KbParamMin=[]  KbParamMax=[]  KtParamMin=[]  KtParamMax=[]  POutMin=[]  POutMax=[]  IOutMin=[]  IOutMax=[]  DOutMin=[]  DOutMax=[]  NOutMin=[]  NOutMax=[]  KbOutMin=[]  KbOutMax=[]  KtOutMin=[]  KtOutMax=[]  IntegratorOutMin=[]  IntegratorOutMax=[]  FilterOutMin=[]  FilterOutMax=[]  SumOutMin=[]  SumOutMax=[]  SumI1OutMin=[]  SumI1OutMax=[]  SumI2OutMin=[]  SumI2OutMax=[]  SumI3OutMin=[]  SumI3OutMax=[]  SumDOutMin=[]  SumDOutMax=[]  SaturationOutMin=[]  SaturationOutMax=[]  IntegratorContinuousStateAttributes=''  IntegratorStateMustResolveToSignalObject=off  IntegratorRTWStateStorageClass=Auto  FilterContinuousStateAttributes=''  FilterStateMustResolveToSignalObject=off  FilterRTWStateStorageClass=Auto  DifferentiatorICPrevScaledInput=0  DifferentiatorOutMin=[]  DifferentiatorOutMax=[]  InitialConditionSetting=State (most efficient)
  PID_from_BJ : simulink/Continuous/PID Controller  Controller=PID  TimeDomain=Discrete-time  SampleTime=0.01  IntegratorMethod=Forward Euler  FilterMethod=Forward Euler  Form=Parallel  UseFilter=on  ControllerParametersSource=internal  P=8.4755768690941  I=0  D=-0.329825259958135  N=18.7162193324192  InitialConditionSource=internal  InitialConditionForIntegrator=0  InitialConditionForFilter=0  ExternalReset=none  LimitOutput=off  UpperSaturationLimit=inf  LowerSaturationLimit=-inf  LinearizeAsGain=off  AntiWindupMode=none  Kb=1  TrackingMode=off  Kt=1  PParamMin=[]  PParamMax=[]  IParamMin=[]  IParamMax=[]  DParamMin=[]  DParamMax=[]  NParamMin=[]  NParamMax=[]  KbParamMin=[]  KbParamMax=[]  KtParamMin=[]  KtParamMax=[]  POutMin=[]  POutMax=[]  IOutMin=[]  IOutMax=[]  DOutMin=[]  DOutMax=[]  NOutMin=[]  NOutMax=[]  KbOutMin=[]  KbOutMax=[]  KtOutMin=[]  KtOutMax=[]  IntegratorOutMin=[]  IntegratorOutMax=[]  FilterOutMin=[]  FilterOutMax=[]  SumOutMin=[]  SumOutMax=[]  SumI1OutMin=[]  SumI1OutMax=[]  SumI2OutMin=[]  SumI2OutMax=[]  SumI3OutMin=[]  SumI3OutMax=[]  SumDOutMin=[]  SumDOutMax=[]  SaturationOutMin=[]  SaturationOutMax=[]  IntegratorContinuousStateAttributes=''  IntegratorStateMustResolveToSignalObject=off  IntegratorRTWStateStorageClass=Auto  FilterContinuousStateAttributes=''  FilterStateMustResolveToSignalObject=off  FilterRTWStateStorageClass=Auto  DifferentiatorICPrevScaledInput=0  DifferentiatorOutMin=[]  DifferentiatorOutMax=[]  InitialConditionSetting=State (most efficient)
  Rate Transition : RateTransition
  Rate Transition1 : RateTransition
  Sum : Sum  Inputs=|+-
  Sum1 : Sum  Inputs=+|+
  DeltaM : Outport
  wires:
  PsiPunktIst/1 -> Sum/2
  PsiPunktSoll/1 -> Sum/1
  Sum/1 -> Rate Transition/1
  2*Jz*rdyn/(br*i)/1 -> Sum1/1
  Manual Switch/1 -> Sum1/2
  Sum1/1 -> Rate Transition1/1
  Rate Transition/1 -> K_OpenLoop1/1, K_ClosedLoop/1
  Rate Transition1/1 -> DeltaM/1
  Constant/1 -> Manual Switch/2
  K_OpenLoop1/1 -> 2*Jz*rdyn/(br*i)/1
  K_ClosedLoop/1 -> PID_fromGA/1
  PID_fromGA/1 -> Manual Switch/1

== system DR18E_Testpult/Verarbeitung/DR18E Torque Control/Torque Filter/PT1 Discrete1/Subsystem ==
  T : Inport
  Constant : Constant
  Constant2 : Constant
  Divide : Product  Inputs=*/
  Divide1 : Product  Inputs=*/
  Sum : Sum  Inputs=|++
  Weighted Sample Time : SampleTimeMath  TsampMathOp=Ts Only
  T* : Outport
  wires:
  Divide1/1 -> Sum/1
  Constant2/1 -> Sum/2
  T/1 -> Divide1/1
  Sum/1 -> Divide/2
  Constant/1 -> Divide/1
  Weighted Sample Time/1 -> Divide1/2
  Divide/1 -> T*/1

== system DR18E_Testpult/Verarbeitung/DR18E Torque Control/Torque Filter/PT1 Discrete3/Subsystem ==
  T : Inport
  Constant : Constant
  Constant2 : Constant
  Divide : Product  Inputs=*/
  Divide1 : Product  Inputs=*/
  Sum : Sum  Inputs=|++
  Weighted Sample Time : SampleTimeMath  TsampMathOp=Ts Only
  T* : Outport
  wires:
  Divide1/1 -> Sum/1
  Constant2/1 -> Sum/2
  T/1 -> Divide1/1
  Sum/1 -> Divide/2
  Constant/1 -> Divide/1
  Weighted Sample Time/1 -> Divide1/2
  Divide/1 -> T*/1

== system DR18E_Testpult/Verarbeitung/Gaspedal Check/PlausibilityCheck/PT1 Discrete/Subsystem ==
  T : Inport
  Constant : Constant
  Constant2 : Constant
  Divide : Product  Inputs=*/
  Divide1 : Product  Inputs=*/
  Sum : Sum  Inputs=|++
  Weighted Sample Time : SampleTimeMath  TsampMathOp=Ts Only
  T* : Outport
  wires:
  Divide1/1 -> Sum/1
  Constant2/1 -> Sum/2
  T/1 -> Divide1/1
  Sum/1 -> Divide/2
  Constant/1 -> Divide/1
  Weighted Sample Time/1 -> Divide1/2
  Divide/1 -> T*/1

== system DR18E_Testpult/Verarbeitung/Gaspedal Check/PlausibilityCheck/PT1 Discrete1/Subsystem ==
  T : Inport
  Constant : Constant
  Constant2 : Constant
  Divide : Product  Inputs=*/
  Divide1 : Product  Inputs=*/
  Sum : Sum  Inputs=|++
  Weighted Sample Time : SampleTimeMath  TsampMathOp=Ts Only
  T* : Outport
  wires:
  Divide1/1 -> Sum/1
  Constant2/1 -> Sum/2
  T/1 -> Divide1/1
  Sum/1 -> Divide/2
  Constant/1 -> Divide/1
  Weighted Sample Time/1 -> Divide1/2
  Divide/1 -> T*/1

== system DR18E_Testpult/Eingabe Fahrzeug/BMS/Voltage 9-10/Voltage Stack 10/RX Timeout Detection/Subsystem ==
  TXStatus : Inport
  Timeout : Inport  Port=2
  Constant : Constant
  Constant1 : Constant  Value=0
  Constant2 : Constant
  Constant3 : Constant  Value=0
  Delay : Delay  DelayLength=1  InitialCondition=0
  Relational Operator : RelationalOperator  Operator=>  OutDataTypeStr=boolean  RndMeth=Nearest
  Sum : Sum  Inputs=|++
  Switch : Switch  Criteria=u2 > Threshold
  Switch1 : Switch  Criteria=u2 > Threshold
  Rampe : Outport
  RX Timeout Error : Outport  Port=2
  wires:
  TXStatus/1 -> Switch/2
  Delay/1 -> Sum/2
  Constant/1 -> Sum/1
  Sum/1 -> Switch/3
  Switch/1 -> Delay/1, Relational Operator/1, Rampe/1
  Constant1/1 -> Switch/1
  Constant2/1 -> Switch1/1
  Constant3/1 -> Switch1/3
  Switch1/1 -> RX Timeout Error/1
  Relational Operator/1 -> Switch1/2
  Timeout/1 -> Relational Operator/2

== system DR18E_Testpult/Eingabe Fahrzeug/BMS/Voltage 9-10/Voltage Stack 10/RX Timeout Detection1/Subsystem ==
  TXStatus : Inport
  Timeout : Inport  Port=2
  Constant : Constant
  Constant1 : Constant  Value=0
  Constant2 : Constant
  Constant3 : Constant  Value=0
  Delay : Delay  DelayLength=1  InitialCondition=0
  Relational Operator : RelationalOperator  Operator=>  OutDataTypeStr=boolean  RndMeth=Nearest
  Sum : Sum  Inputs=|++
  Switch : Switch  Criteria=u2 > Threshold
  Switch1 : Switch  Criteria=u2 > Threshold
  Rampe : Outport
  RX Timeout Error : Outport  Port=2
  wires:
  TXStatus/1 -> Switch/2
  Delay/1 -> Sum/2
  Constant/1 -> Sum/1
  Sum/1 -> Switch/3
  Switch/1 -> Delay/1, Relational Operator/1, Rampe/1
  Constant1/1 -> Switch/1
  Constant2/1 -> Switch1/1
  Constant3/1 -> Switch1/3
  Switch1/1 -> RX Timeout Error/1
  Relational Operator/1 -> Switch1/2
  Timeout/1 -> Relational Operator/2

== system DR18E_Testpult/Eingabe Fahrzeug/BMS/Voltage 9-10/Voltage Stack 10/RX Timeout Detection2/Subsystem ==
  TXStatus : Inport
  Timeout : Inport  Port=2
  Constant : Constant
  Constant1 : Constant  Value=0
  Constant2 : Constant
  Constant3 : Constant  Value=0
  Delay : Delay  DelayLength=1  InitialCondition=0
  Relational Operator : RelationalOperator  Operator=>  OutDataTypeStr=boolean  RndMeth=Nearest
  Sum : Sum  Inputs=|++
  Switch : Switch  Criteria=u2 > Threshold
  Switch1 : Switch  Criteria=u2 > Threshold
  Rampe : Outport
  RX Timeout Error : Outport  Port=2
  wires:
  TXStatus/1 -> Switch/2
  Delay/1 -> Sum/2
  Constant/1 -> Sum/1
  Sum/1 -> Switch/3
  Switch/1 -> Delay/1, Relational Operator/1, Rampe/1
  Constant1/1 -> Switch/1
  Constant2/1 -> Switch1/1
  Constant3/1 -> Switch1/3
  Switch1/1 -> RX Timeout Error/1
  Relational Operator/1 -> Switch1/2
  Timeout/1 -> Relational Operator/2

== system DR18E_Testpult/Eingabe Fahrzeug/BMS/Voltage 9-10/Voltage Stack 9/RX Timeout Detection/Subsystem ==
  TXStatus : Inport
  Timeout : Inport  Port=2
  Constant : Constant
  Constant1 : Constant  Value=0
  Constant2 : Constant
  Constant3 : Constant  Value=0
  Delay : Delay  DelayLength=1  InitialCondition=0
  Relational Operator : RelationalOperator  Operator=>  OutDataTypeStr=boolean  RndMeth=Nearest
  Sum : Sum  Inputs=|++
  Switch : Switch  Criteria=u2 > Threshold
  Switch1 : Switch  Criteria=u2 > Threshold
  Rampe : Outport
  RX Timeout Error : Outport  Port=2
  wires:
  TXStatus/1 -> Switch/2
  Delay/1 -> Sum/2
  Constant/1 -> Sum/1
  Sum/1 -> Switch/3
  Switch/1 -> Delay/1, Relational Operator/1, Rampe/1
  Constant1/1 -> Switch/1
  Constant2/1 -> Switch1/1
  Constant3/1 -> Switch1/3
  Switch1/1 -> RX Timeout Error/1
  Relational Operator/1 -> Switch1/2
  Timeout/1 -> Relational Operator/2

== system DR18E_Testpult/Eingabe Fahrzeug/BMS/Voltage 9-10/Voltage Stack 9/RX Timeout Detection1/Subsystem ==
  TXStatus : Inport
  Timeout : Inport  Port=2
  Constant : Constant
  Constant1 : Constant  Value=0
  Constant2 : Constant
  Constant3 : Constant  Value=0
  Delay : Delay  DelayLength=1  InitialCondition=0
  Relational Operator : RelationalOperator  Operator=>  OutDataTypeStr=boolean  RndMeth=Nearest
  Sum : Sum  Inputs=|++
  Switch : Switch  Criteria=u2 > Threshold
  Switch1 : Switch  Criteria=u2 > Threshold
  Rampe : Outport
  RX Timeout Error : Outport  Port=2
  wires:
  TXStatus/1 -> Switch/2
  Delay/1 -> Sum/2
  Constant/1 -> Sum/1
  Sum/1 -> Switch/3
  Switch/1 -> Delay/1, Relational Operator/1, Rampe/1
  Constant1/1 -> Switch/1
  Constant2/1 -> Switch1/1
  Constant3/1 -> Switch1/3
  Switch1/1 -> RX Timeout Error/1
  Relational Operator/1 -> Switch1/2
  Timeout/1 -> Relational Operator/2

== system DR18E_Testpult/Eingabe Fahrzeug/BMS/Voltage 9-10/Voltage Stack 9/RX Timeout Detection2/Subsystem ==
  TXStatus : Inport
  Timeout : Inport  Port=2
  Constant : Constant
  Constant1 : Constant  Value=0
  Constant2 : Constant
  Constant3 : Constant  Value=0
  Delay : Delay  DelayLength=1  InitialCondition=0
  Relational Operator : RelationalOperator  Operator=>  OutDataTypeStr=boolean  RndMeth=Nearest
  Sum : Sum  Inputs=|++
  Switch : Switch  Criteria=u2 > Threshold
  Switch1 : Switch  Criteria=u2 > Threshold
  Rampe : Outport
  RX Timeout Error : Outport  Port=2
  wires:
  TXStatus/1 -> Switch/2
  Delay/1 -> Sum/2
  Constant/1 -> Sum/1
  Sum/1 -> Switch/3
  Switch/1 -> Delay/1, Relational Operator/1, Rampe/1
  Constant1/1 -> Switch/1
  Constant2/1 -> Switch1/1
  Constant3/1 -> Switch1/3
  Switch1/1 -> RX Timeout Error/1
  Relational Operator/1 -> Switch1/2
  Timeout/1 -> Relational Operator/2

== system DR18E_Testpult/Eingabe Fahrzeug/BMS/Voltage Stack 1-2/Voltage Stack 1/RX Timeout Detection/Subsystem ==
  TXStatus : Inport
  Timeout : Inport  Port=2
  Constant : Constant
  Constant1 : Constant  Value=0
  Constant2 : Constant
  Constant3 : Constant  Value=0
  Delay : Delay  DelayLength=1  InitialCondition=0
  Relational Operator : RelationalOperator  Operator=>  OutDataTypeStr=boolean  RndMeth=Nearest
  Sum : Sum  Inputs=|++
  Switch : Switch  Criteria=u2 > Threshold
  Switch1 : Switch  Criteria=u2 > Threshold
  Rampe : Outport
  RX Timeout Error : Outport  Port=2
  wires:
  TXStatus/1 -> Switch/2
  Delay/1 -> Sum/2
  Constant/1 -> Sum/1
  Sum/1 -> Switch/3
  Switch/1 -> Delay/1, Relational Operator/1, Rampe/1
  Constant1/1 -> Switch/1
  Constant2/1 -> Switch1/1
  Constant3/1 -> Switch1/3
  Switch1/1 -> RX Timeout Error/1
  Relational Operator/1 -> Switch1/2
  Timeout/1 -> Relational Operator/2

== system DR18E_Testpult/Eingabe Fahrzeug/BMS/Voltage Stack 1-2/Voltage Stack 1/RX Timeout Detection1/Subsystem ==
  TXStatus : Inport
  Timeout : Inport  Port=2
  Constant : Constant
  Constant1 : Constant  Value=0
  Constant2 : Constant
  Constant3 : Constant  Value=0
  Delay : Delay  DelayLength=1  InitialCondition=0
  Relational Operator : RelationalOperator  Operator=>  OutDataTypeStr=boolean  RndMeth=Nearest
  Sum : Sum  Inputs=|++
  Switch : Switch  Criteria=u2 > Threshold
  Switch1 : Switch  Criteria=u2 > Threshold
  Rampe : Outport
  RX Timeout Error : Outport  Port=2
  wires:
  TXStatus/1 -> Switch/2
  Delay/1 -> Sum/2
  Constant/1 -> Sum/1
  Sum/1 -> Switch/3
  Switch/1 -> Delay/1, Relational Operator/1, Rampe/1
  Constant1/1 -> Switch/1
  Constant2/1 -> Switch1/1
  Constant3/1 -> Switch1/3
  Switch1/1 -> RX Timeout Error/1
  Relational Operator/1 -> Switch1/2
  Timeout/1 -> Relational Operator/2

== system DR18E_Testpult/Eingabe Fahrzeug/BMS/Voltage Stack 1-2/Voltage Stack 1/RX Timeout Detection2/Subsystem ==
  TXStatus : Inport
  Timeout : Inport  Port=2
  Constant : Constant
  Constant1 : Constant  Value=0
  Constant2 : Constant
  Constant3 : Constant  Value=0
  Delay : Delay  DelayLength=1  InitialCondition=0
  Relational Operator : RelationalOperator  Operator=>  OutDataTypeStr=boolean  RndMeth=Nearest
  Sum : Sum  Inputs=|++
  Switch : Switch  Criteria=u2 > Threshold
  Switch1 : Switch  Criteria=u2 > Threshold
  Rampe : Outport
  RX Timeout Error : Outport  Port=2
  wires:
  TXStatus/1 -> Switch/2
  Delay/1 -> Sum/2
  Constant/1 -> Sum/1
  Sum/1 -> Switch/3
  Switch/1 -> Delay/1, Relational Operator/1, Rampe/1
  Constant1/1 -> Switch/1
  Constant2/1 -> Switch1/1
  Constant3/1 -> Switch1/3
  Switch1/1 -> RX Timeout Error/1
  Relational Operator/1 -> Switch1/2
  Timeout/1 -> Relational Operator/2

== system DR18E_Testpult/Eingabe Fahrzeug/BMS/Voltage Stack 1-2/Voltage Stack 2/RX Timeout Detection/Subsystem ==
  TXStatus : Inport
  Timeout : Inport  Port=2
  Constant : Constant
  Constant1 : Constant  Value=0
  Constant2 : Constant
  Constant3 : Constant  Value=0
  Delay : Delay  DelayLength=1  InitialCondition=0
  Relational Operator : RelationalOperator  Operator=>  OutDataTypeStr=boolean  RndMeth=Nearest
  Sum : Sum  Inputs=|++
  Switch : Switch  Criteria=u2 > Threshold
  Switch1 : Switch  Criteria=u2 > Threshold
  Rampe : Outport
  RX Timeout Error : Outport  Port=2
  wires:
  TXStatus/1 -> Switch/2
  Delay/1 -> Sum/2
  Constant/1 -> Sum/1
  Sum/1 -> Switch/3
  Switch/1 -> Delay/1, Relational Operator/1, Rampe/1
  Constant1/1 -> Switch/1
  Constant2/1 -> Switch1/1
  Constant3/1 -> Switch1/3
  Switch1/1 -> RX Timeout Error/1
  Relational Operator/1 -> Switch1/2
  Timeout/1 -> Relational Operator/2

== system DR18E_Testpult/Eingabe Fahrzeug/BMS/Voltage Stack 1-2/Voltage Stack 2/RX Timeout Detection1/Subsystem ==
  TXStatus : Inport
  Timeout : Inport  Port=2
  Constant : Constant
  Constant1 : Constant  Value=0
  Constant2 : Constant
  Constant3 : Constant  Value=0
  Delay : Delay  DelayLength=1  InitialCondition=0
  Relational Operator : RelationalOperator  Operator=>  OutDataTypeStr=boolean  RndMeth=Nearest
  Sum : Sum  Inputs=|++
  Switch : Switch  Criteria=u2 > Threshold
  Switch1 : Switch  Criteria=u2 > Threshold
  Rampe : Outport
  RX Timeout Error : Outport  Port=2
  wires:
  TXStatus/1 -> Switch/2
  Delay/1 -> Sum/2
  Constant/1 -> Sum/1
  Sum/1 -> Switch/3
  Switch/1 -> Delay/1, Relational Operator/1, Rampe/1
  Constant1/1 -> Switch/1
  Constant2/1 -> Switch1/1
  Constant3/1 -> Switch1/3
  Switch1/1 -> RX Timeout Error/1
  Relational Operator/1 -> Switch1/2
  Timeout/1 -> Relational Operator/2
